simulink model "stepper_control"  (R2022a)
settings: Solver=FixedStepAuto  StartTime=0.0  StopTime=inf  FixedStep=0.00005  RelTol=1e-3
libraries: arduinolib x18, simulink x8, robotcorelib x2
settings Model: FPTRunName=Active  ExtModeTrigDuration=2  Creator=The MathWorks, Inc.  LastModifiedBy=15031
settings SolverCC: AlgebraicLoopSolver=TrustRegion
settings DataIOCC: LimitDataPoints=on  ReturnWorkspaceOutputs=off
settings OptimizationCC: ExpressionDepthLimit=2147483647  LifeSpan=Inf  MaxStackSize=64
settings DebuggingCC: UnderspecifiedInitializationDetection=Classic  MergeDetectMultiDrivingBlocksExec=none  FcnCallInpInsideContextMsg=warning  UnconnectedInputMsg=warning  UnconnectedOutputMsg=warning  UnconnectedLineMsg=warning  AllowSymbolicDim=off  StateNameClashWarn=warning  SFUnexpectedBacktrackingDiag=warning  SFNoUnconditionalDefaultTransitionDiag=warning  SFExecutionAtInitializationDiag=none  SFMachineParentedDataDiag=warning  ArithmeticOperatorsInVariantConditions=warning
settings HardwareCC: ProdBitPerInt=16  ProdBitPerPointer=16  ProdBitPerSizeT=16  ProdBitPerPtrDiffT=16  ProdLargestAtomicFloat=None  ProdWordSize=8  ProdHWDeviceType=Atmel->AVR  UseEmbeddedCoderFeatures=off  UseSimulinkCoderFeatures=off
settings ModelReferenceCC: PropagateSignalLabelsOutOfModel=off
settings SFSimCC: SimUseLocalCustomCode=off  MATLABDynamicMemAlloc=off
settings RTWCC: SystemTargetFile=ert.tlc  HardwareBoard=Arduino Mega 2560  TemplateMakefile=ert_default_tmf  GenerateReport=on  RTWVerbose=off  RTWUseLocalCustomCode=off  Toolchain=Arduino AVR  BuildConfiguration=Faster Runs  LaunchReport=on  DLArmComputeVersion=19.05
settings CodeAppCC: ForceParamTrailComments=on  OperatorAnnotations=on  StateflowObjectComments=on  MATLABSourceComments=on
settings ERTTargetCC: MultiwordLength=2048  ERTCustomFileBanners=off  SupportContinuousTime=on  SupportNonInlinedSFcns=on  RemoveResetFunc=off  ModelStepFunctionPrototypeControlCompliant=off
settings ConfigComp: CovMetricSettings=dw  CovSaveCumulativeToWorkspaceVar=on  CovSaveSingleToWorkspaceVar=on  CovExternalEMLEnable=off  CovSFcnEnable=off

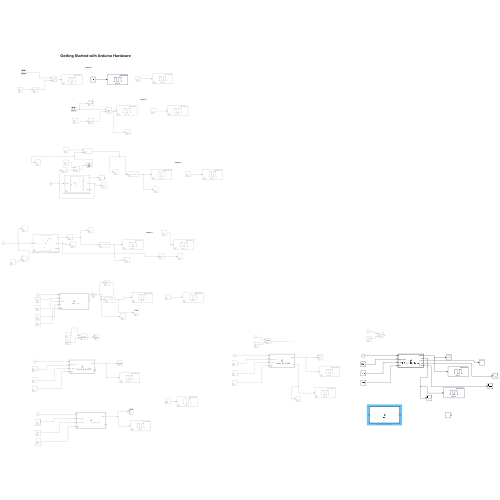
[thumbnail: Simulink's stored preview of the top-level diagram]
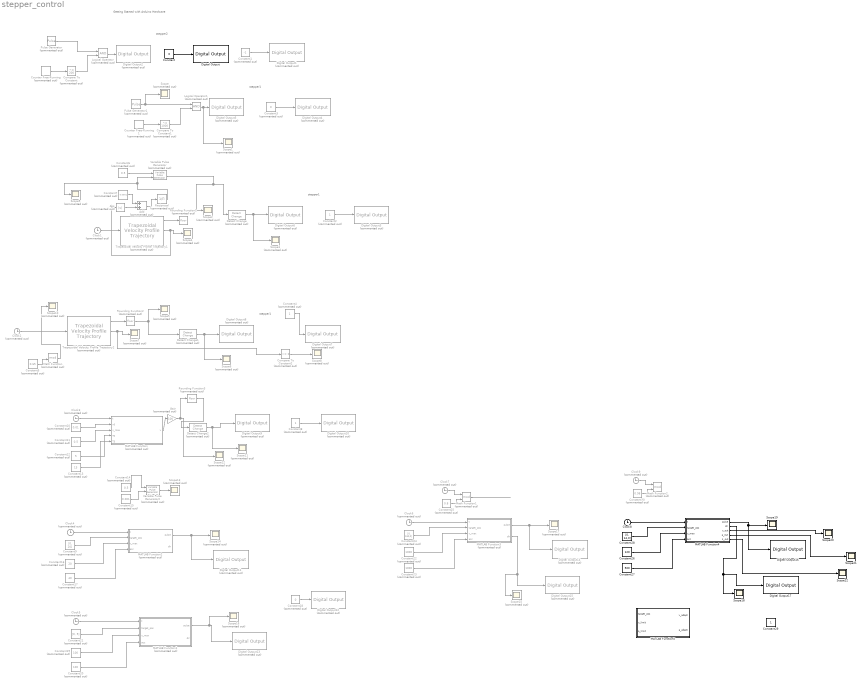
== system stepper_control ==
  note: stepper2
  note: Getting Started with Arduino Hardware
  note: stepper1
  note: stepper1
  note: stepper1
  Abs : Abs  Commented=on  SaturateOnIntegerOverflow=off
  Add : Sum  Commented=on
  Clock{1..7,9} (8 alike) : Clock  Commented=on
  Clock8 : Clock
  Compare To Constant : simulink/Logic and Bit Operations/Compare To Constant  Commented=on  relop=<=  const=200  OutDataTypeStr=boolean
  Compare To Constant1 : simulink/Logic and Bit Operations/Compare To Constant  Commented=on  relop=<=  const=1000  OutDataTypeStr=boolean
  Compare To Constant2 : simulink/Logic and Bit Operations/Compare To Constant  Commented=on  relop=>=  const=0  OutDataTypeStr=uint8
  Constant : Constant  Value=0
  Constant1 : Constant  Commented=on  Value=-1
  Constant10 : Constant  Commented=on  Value=0.01
  Constant11 : Constant  Commented=on  Value=0.5
  Constant12 : Constant  Commented=on  Value=5
  Constant13 : Constant  Commented=on  Value=13
  Constant14 : Constant  Commented=on  Value=0.5
  Constant15 : Constant  Commented=on  Value=0.001
  Constant16 : Constant  Commented=on  Value=20
  Constant17 : Constant  Commented=on  Value=40
  Constant18 : Constant  Commented=on  Value=0
  Constant19 : Constant  Commented=on  Value=100
  Constant2 : Constant  Commented=on
  Constant20 : Constant  Commented=on  Value=100
  Constant21 : Constant  Commented=on  Value=[0, 5]
  Constant22 : Constant  Commented=on  Value=1000
  Constant23 : Constant  Commented=on  Value=1000
  Constant24 : Constant  Commented=on  Value=[0, 240,0]
  Constant25 : Constant  Commented=on  Value=0.8
  Constant26 : Constant  Value=120
  Constant27 : Constant  Value=500
  Constant28 : Constant  Value=[0, 14,0]
  Constant29 : Constant
  Constant3 : Constant  Commented=on  Value=0
  Constant30 : Constant  Commented=on  Value=0.98
  Constant4 : Constant  Commented=on
  Constant5 : Constant  Commented=on  Value=0.65
  Constant6 : Constant  Commented=on  Value=0.5
  Constant7 : Constant  Commented=on  Value=0.0001
  Constant8 : Constant  Commented=on
  Constant9 : Constant  Commented=on  Value=[0, 20]
  Counter Free-Running : simulink/Sources/Counter Free-Running  Commented=on  NumBits=32  tsamp=0.002
  Counter Free-Running1 : simulink/Sources/Counter Free-Running  Commented=on  NumBits=32  tsamp=0.0002
  Detect Change : simulink/Logic and Bit Operations/Detect Change  Commented=on  vinit=0  OutDataTypeStr=uint8
  Detect Change1 : simulink/Logic and Bit Operations/Detect Change  Commented=on  vinit=0  InputProcessing=Columns as channels (frame based)  OutDataTypeStr=uint8
  Detect Change2 : simulink/Logic and Bit Operations/Detect Change  Commented=on  vinit=0  InputProcessing=Columns as channels (frame based)  OutDataTypeStr=uint8
  Digital Output : arduinolib/Digital Output  pinNumber=8  Direction=output  blockPlatform=arduino
  Digital Output{1,7,10,12} (4 alike) : arduinolib/Digital Output  Commented=on  pinNumber=6  Direction=output  blockPlatform=arduino
  Digital Output{2,8..9,11,13} (5 alike) : arduinolib/Digital Output  Commented=on  pinNumber=3  Direction=output  blockPlatform=arduino
  Digital Output14 : arduinolib/Digital Output  Commented=on  pinNumber=4  Direction=output  blockPlatform=arduino
  Digital Output15 : arduinolib/Digital Output  Commented=on  pinNumber=7  Direction=output  blockPlatform=arduino
  Digital Output16 : arduinolib/Digital Output  pinNumber=3  Direction=output  blockPlatform=arduino
  Digital Output17 : arduinolib/Digital Output  pinNumber=6  Direction=output  blockPlatform=arduino
  Digital Output3 : arduinolib/Digital Output  Commented=on  pinNumber=7  Direction=output  blockPlatform=arduino
  Digital Output4 : arduinolib/Digital Output  Commented=on  pinNumber=7  Direction=output  blockPlatform=arduino
  Digital Output5 : arduinolib/Digital Output  Commented=on  pinNumber=4  Direction=output  blockPlatform=arduino
  Digital Output6 : arduinolib/Digital Output  Commented=on  pinNumber=4  Direction=output  blockPlatform=arduino
  Gain : Gain  Commented=on  Gain=100
  Logical Operator : Logic  Commented=on  AllPortsSameDT=off  OutDataTypeStr=boolean
  Logical Operator1 : Logic  Commented=on  AllPortsSameDT=off  OutDataTypeStr=boolean
  MATLAB Function : MATLAB Function  Commented=on  TreatAsAtomicUnit=on
  MATLAB Function1 : MATLAB Function  Commented=on  TreatAsAtomicUnit=on
  MATLAB Function2 : MATLAB Function  Commented=on  TreatAsAtomicUnit=on
  MATLAB Function3 : MATLAB Function  Commented=on  TreatAsAtomicUnit=on
  MATLAB Function4 : MATLAB Function  TreatAsAtomicUnit=on
  MATLAB Function5 : MATLAB Function  TreatAsAtomicUnit=on
  Math Function : Math  Commented=on  Operator=mod
  Math Function1 : Math  Commented=on  Operator=mod
  Math Function2 : Math  Commented=on  Operator=mod
  Pulse Generator : DiscretePulseGenerator  Commented=on  SampleTime=0.001
  Pulse Generator1 : DiscretePulseGenerator  Commented=on  SampleTime=0.0001
  Reciprocal : Product  Commented=on  Inputs=/
  Rounding Function1 : Rounding  Commented=on
  Rounding Function2 : Rounding  Commented=on
  Rounding Function3 : Rounding  Commented=on
  Scope{,1..17} (18 alike) : Scope  Commented=on
  Scope{18..22} (5 alike) : Scope
  Trapezoidal Velocity Profile Trajectory1 : robotcorelib/Trapezoidal Velocity Profile Trajectory  Commented=on  WaypointSource=Internal  Waypoints=[0,2000]  NumParams=2  Parameter1=Acceleration  Parameter2=Peak Velocity  ParameterSource=Internal  PeakVelocity=5000  Acceleration=30000  EndTime=[ 1; 1 ]  AccelTime=[0,3 ]  SimulateUsing=Interpreted execution
      settings: SourceProductBaseCode=RO,NV,RR,UV
  Trapezoidal Velocity Profile Trajectory2 : robotcorelib/Trapezoidal Velocity Profile Trajectory  Commented=on  WaypointSource=Internal  Waypoints=[0,2300,0]  NumParams=2  Parameter1=Acceleration  Parameter2=Peak Velocity  ParameterSource=Internal  PeakVelocity=12000  Acceleration=100000  EndTime=[ 1; 1 ]  AccelTime=[0,3 ]  SimulateUsing=Interpreted execution
      settings: SourceProductBaseCode=RO,NV,RR,UV
  Variable Pulse Generator : VariablePulseGenerator  Commented=on  RunAtFixedTimeIntervals=on  SampleTime=0.0001
  Variable Pulse Generator2 : VariablePulseGenerator  Commented=on  AllowZeroPulseWidth=on  RunAtFixedTimeIntervals=on  SampleTime=0.00005
  wires:
  Pulse Generator/1 -> Logical Operator/1
  Constant/1 -> Digital Output/1
  Constant1/1 -> Digital Output1/1
  Compare To Constant/1 -> Logical Operator/2
  Logical Operator/1 -> Digital Output2/1
  Counter Free-Running/1 -> Compare To Constant/1
  Logical Operator1/1 -> Scope1/1, Digital Output5/1
  Pulse Generator1/1 -> Logical Operator1/1, Scope/1
  Counter Free-Running1/1 -> Compare To Constant1/1
  Compare To Constant1/1 -> Logical Operator1/2
  Constant3/1 -> Digital Output4/1
  Clock1/1 -> Trapezoidal Velocity Profile Trajectory1/1
  Constant2/1 -> Digital Output3/1
  Trapezoidal Velocity Profile Trajectory1/1 -> Rounding Function1/1
  Variable Pulse Generator/1 -> Scope2/1, Detect Change/1
  Trapezoidal Velocity Profile Trajectory1/2 -> Abs/1, Scope4/1
  Trapezoidal Velocity Profile Trajectory2/2 -> Compare To Constant2/1, Scope7/1
  Trapezoidal Velocity Profile Trajectory2/1 -> Rounding Function2/1
  Detect Change1/1 -> Scope6/1, Digital Output8/1
  Compare To Constant2/1 -> Scope8/1
  Rounding Function2/1 -> Scope5/1, Detect Change1/1
  Constant5/1 -> Math Function/2
  Detect Change/1 -> Scope3/1, Digital Output6/1
  Constant6/1 -> Variable Pulse Generator/1
  Abs/1 -> Add/2
  Reciprocal/1 -> Scope9/1, Variable Pulse Generator/2
  Add/1 -> Reciprocal/1
  Constant7/1 -> Add/1
  Clock2/1 -> Trapezoidal Velocity Profile Trajectory2/1
  Math Function/1 -> Scope10/1
  Clock3/1 -> MATLAB Function/1(t)
  Constant8/1 -> Digital Output10/1
  Constant10/1 -> MATLAB Function/2(v0)
  Constant11/1 -> MATLAB Function/3(v_max)
  Constant12/1 -> MATLAB Function/4(T0)
  Constant13/1 -> MATLAB Function/5(T3)
  Constant14/1 -> Variable Pulse Generator2/1
  Constant15/1 -> Variable Pulse Generator2/2
  Variable Pulse Generator2/1 -> Scope13/1
  Detect Change2/1 -> Scope11/1, Digital Output9/1
  MATLAB Function/1(v) -> Gain/1
  Gain/1 -> Rounding Function3/1, Scope12/1
  Rounding Function3/1 -> Detect Change2/1
  Constant17/1 -> MATLAB Function2/4(acc)
  Clock4/1 -> MATLAB Function2/1(t)
  Constant9/1 -> MATLAB Function2/2(target_pos)
  Constant16/1 -> MATLAB Function2/3(v_max)
  MATLAB Function2/1(pulse) -> Digital Output11/1, Scope14/1
  Constant4/1 -> Digital Output7/1
  Constant18/1 -> Digital Output12/1
  Constant21/1 -> MATLAB Function1/2(target_pos)
  Constant19/1 -> MATLAB Function1/3(v_max)
  Constant20/1 -> MATLAB Function1/4(acc)
  Clock5/1 -> MATLAB Function1/1(t)
  MATLAB Function1/1(pulse) -> Scope16/1, Digital Output13/1
  Constant24/1 -> MATLAB Function3/2(target_pos)
  Constant22/1 -> MATLAB Function3/3(v_max)
  MATLAB Function3/1(pulse) -> Digital Output14/1, Scope17/1
  Constant23/1 -> MATLAB Function3/4(acc)
  Clock6/1 -> MATLAB Function3/1(t)
  Constant25/1 -> Math Function1/2
  Math Function1/1 -> ?
  Clock7/1 -> Math Function1/1
  MATLAB Function3/2(dir) -> Digital Output15/1, Scope15/1
  Constant26/1 -> MATLAB Function4/3(v_max)
  Constant28/1 -> MATLAB Function4/2(target_pos)
  MATLAB Function4/2(dir) -> Scope18/1, Digital Output17/1
  MATLAB Function4/1(pulse) -> Digital Output16/1, Scope19/1
  Constant27/1 -> MATLAB Function4/4(acc)
  Constant30/1 -> Math Function2/2
  Clock9/1 -> Math Function2/1
  Clock8/1 -> MATLAB Function4/1(t)
  MATLAB Function4/3(v_out) -> Scope20/1
  MATLAB Function4/4(a_out) -> Scope21/1
  MATLAB Function4/5(s_out) -> Scope22/1

== matlab function stepper_control/MATLAB Function1 ==
  data: t input; pulse output; target_pos input; v_max input; acc input; dir output
function [pulse, dir] = S_Trapezoidal_Control(t, target_pos, v_max, acc)
    % 硬件常数定义 [cite: 73]
    K = 160; % 脉冲/mm [cite: 73]
    
    % 使用 persistent 变量存储状态，模仿单片机寄存器 [cite: 84, 125]
    persistent idx              % 当前目标点索引
    persistent startTime        % 当前路段起始时间
    persistent last_toggle_time % 上次脉冲翻转时间
    persistent current_state    % 当前脉冲电平状态
    
    % 初始化 [cite: 86]
    if isempty(idx)
        idx = 2; % 从 Waypoints 的第二个元素开始 (0 -> 2300)
        startTime = 0;
        last_toggle_time = 0;
        current_state = 0;
    end

    % --- 阶段 1: 轨迹规划与目标点切换 ---
    current_target = target_pos(idx);
    previous_target = target_pos(idx-1);
    S_total = abs(current_target - previous_target); % 本段总位移 [cite: 77]
    
    % 计算本段运行时间 (简化版 S-梯形时间分配) [cite: 23]
    % 注意：实际算法中 T0 需根据 S_total 校验，防止位移太短达不到 v_max [cite: 207]
    T_acc = 1.5 * (v_max / acc); % 加速阶段总长 [cite: 23, 210]
    T_const = S_total / v_max - T_acc; % 匀速阶段时长 [cite: 79]
    if T_const < 0, T_const = 0; end % 防错处理
    
    dt = t - startTime; % 本段已运行时间
    
    % 速度 v 计算 (根据论文公式 3 实现) [cite: 38, 72]
    T0 = v_max / (acc * 0.75); % 加加速特征时间 [cite: 23]
    if dt < T0
        v = 0.5 * (acc/T0) * dt^2; % 加加速 [cite: 31, 41]
    elseif dt < 1.5 * T0
        v = 0.5 * acc * T0 + acc * (dt - T0); % 匀加速 [cite: 36, 42]
    elseif dt < (1.5 * T0 + T_const)
        v = v_max; % 匀速 [cite: 32, 43]
    elseif dt < (3.0 * T0 + T_const)
        % 减速逻辑 (镜像加速过程) [cite: 23, 63]
        d_dt = (3.0 * T0 + T_const) - dt;
        v = 0.5 * (acc/T0) * d_dt^2;
    else
        v = 0;
        % 判定到达，切换到下一个路标点 
        if idx < length(target_pos)
            idx = idx + 1;
            startTime = t;
        end
    end

    % --- 阶段 2: 脉冲产生逻辑 --- [cite: 125]
    if v > 0.01
        T_pulse = 1 / (K * v); % 计算脉冲周期 [cite: 75]
        % 频率翻转逻辑 [cite: 102]
        if (t - last_toggle_time) >= (T_pulse / 2)
            current_state = 1 - current_state;
            last_toggle_time = t;
        end
    else
        current_state = 0;
    end

    % --- 阶段 3: 确定输出 (强制标量输出以防 Arduino 报错) ---
    pulse = double(current_state); % 必须是单个数值
    % 方向判定：根据当前目标与前一目标的差值确定 [cite: 21, 240]
    if current_target >= previous_target
        dir = 1.0; 
    else
        dir = 0.0;
    end
end

== matlab function stepper_control/MATLAB Function ==
  data: t input; v output; v0 input; v_max input; T0 input; T3 input
function v  = S_Curve_Gen(t, v0, v_max, T0, T3)
    % t: 当前仿真时间
    % v0: 启动速度
    % v_max: 设定运行速度 (Vh)
    % T0: 代数常数，用于确定加减速阶段时长 (根据论文 T_acc = 1.5*T0)
    % T3: 匀速阶段持续时间

    J = (v_max - v0) / (1.25 * T0^2); % 根据公式(3)推导的加加速度 J
    
    % 阶段时间节点定义 [cite: 23, 54]
    t1 = T0;               % 加加速结束
    t2 = 1.5 * T0;         % 匀加速结束（达到设定速度）
    t3 = t2 + T3;          % 匀速结束
    t4 = t3 + 0.5 * T0;    % 匀减速结束
    t5 = t3 + 1.5 * T0;    % 减减速结束（停止）

    if t >= 0 && t < t1
        % 加加速阶段 [cite: 31, 41]
        v = v0 + 0.5 * J * t^2;
    elseif t >= t1 && t < t2
        % 匀加速阶段 [cite: 36, 42]
        v = v0 - 0.5 * J * T0^2 + J * T0 * t;
    elseif t >= t2 && t < t3
        % 匀速阶段 [cite: 32, 43]
        v = v_max;
    elseif t >= t3 && t < t4
        % 匀减速阶段 [cite: 40, 44]
        v = v_max + 2.5 * J * T0^2 - J * T0 * (t - t3); % 参考公式(3)减速逻辑
    elseif t >= t4 && t <= t5
        % 减减速阶段 [cite: 69]
        % 此处根据公式(3)最后一段逻辑实现平滑减速至v0
        dt = t5 - t;
        v = v0 + 0.5 * J * dt^2;
    else
        v = 0; % 运行结束
    end
end

== matlab function stepper_control/MATLAB Function2 ==
  data: t input; pulse output; target_pos input; v_max input; acc input; dir output
function [pulse, dir] = S_Trapezoidal_Control(t, target_pos, v_max, acc)
    % 硬件常数：160 脉冲/mm
    K = 160; 
    
    % 持久变量：模拟单片机寄存器
    persistent idx startTime last_toggle_time current_state
    persistent T_acc T_const T_dec v_peak current_dist
    
    num_points = length(target_pos); 

    % 1. 初始化逻辑
    if isempty(idx)
        idx = 2; 
        startTime = 0;
        last_toggle_time = 0;
        current_state = 0;
        current_dist = 0; 
        
        % 初始化第一段参数
        p1 = target_pos(1);
        p2 = target_pos(min(idx, num_points));
        [T_acc, T_const, T_dec, v_peak] = calc_params(p1, p2, v_max, acc);
    end

    % 2. 确定当前参考点和总位移
    curr_idx = min(idx, num_points);
    prev_idx = max(1, curr_idx - 1);
    S_total = abs(target_pos(curr_idx) - target_pos(prev_idx)); 
    
    dt = t - startTime;
    T0 = v_peak / (acc * 0.75); % S曲线特征时间点 (加加速结束点)
    
    % 关键：定义完整的减速结束时间 T_end
    % S曲线对称性：加速耗时 1.5*T0, 减速耗时 1.5*T0
    T_end = 1.5*T0 + T_const + 1.5*T0;

    % --- 阶段 1: 速度规划与逻辑切换 ---
    if dt >= T_end || (current_dist >= S_total && S_total > 0 && dt > T_end*0.8)
        v = 0;
        % 到达终点，尝试切换到下一个路标
        if idx < num_points
            idx = idx + 1;
            startTime = t;
            current_dist = 0; 
            [T_acc, T_const, T_dec, v_peak] = calc_params(target_pos(idx-1), target_pos(idx), v_max, acc);
        end
    else
        % --- S-梯形速度分段函数 (核心修正) ---
        if dt < T0
            % 阶段1: 加加速 (速度按二次方上升)
            v = 0.5 * (acc/T0) * dt^2;
        elseif dt < 1.5 * T0
            % 阶段2: 匀加速 (速度线性上升)
            v = 0.5 * acc * T0 + acc * (dt - T0);
        elseif dt < (1.5 * T0 + T_const)
            % 阶段3: 匀速
            v = v_peak;
        elseif dt < (3.0 * T0 + T_const)
            % 阶段4: 减速 (镜像加速阶段，确保波形平滑变稀疏)
            % 计算距离终点的剩余时间 d_dt
            d_dt = (3.0 * T0 + T_const) - dt;
            if d_dt < 0, d_dt = 0; end
            v = 0.5 * (acc/T0) * d_dt^2; 
        else
            v = 0; 
        end
    end

    % --- 阶段 2: 脉冲翻转与位移累加 ---
    if v > 0.05
        T_period = 1 / (K * v); 
        if (t - last_toggle_time) >= (T_period / 2)
            current_state = 1 - current_state;
            last_toggle_time = t;
            % 仅在上升沿累加位移，保证精度
            if current_state == 1
                current_dist = current_dist + (1 / K);
            end
        end
    else
        current_state = 0;
    end

    % --- 阶段 3: 输出信号 ---
    pulse = double(current_state);
    if target_pos(curr_idx) >= target_pos(prev_idx)
        dir = 1.0; 
    else
        dir = 0.0;
    end
end

% 辅助函数：路段参数计算
function [Ta, Tc, Td, vp] = calc_params(p1, p2, vmax, a)
    dist = abs(p2 - p1);
    if dist < 1e-5, dist = 1e-5; end
    
    % 计算达到最大速度所需的最小距离 (S曲线加速+减速)
    S_acc_limit = 1.5 * (vmax^2 / a); 
    
    if dist >= S_acc_limit
        vp = vmax;
        Ta = 1.5 * (vmax / a);
        Tc = (dist - S_acc_limit) / vmax;
    else
        % 距离不足时，通过降速保证完整的S形起停
        vp = sqrt(dist * a / 1.5); 
        Ta = 1.5 * (vp / a);
        Tc = 0;
    end
    Td = Ta;
end

== matlab function stepper_control/MATLAB Function3 ==
  data: t input; pulse output; target_pos input; v_max input; acc input; dir output
function [pulse, dir] = S_Trapezoidal_Control(t, target_pos, v_max, acc)
    K = 160; % 160 pulses/mm
    persistent idx startTime last_toggle_time current_state current_dist
    persistent T_acc T_const v_peak
    
    num_pts = length(target_pos);
    if isempty(idx)
        idx = 2; startTime = 0; last_toggle_time = 0;
        current_state = 0; current_dist = 0;
        [T_acc, T_const, v_peak] = calc_logic(target_pos(1), target_pos(2), v_max, acc);
    end

    dt = t - startTime;
    S_total = abs(target_pos(idx) - target_pos(idx-1));
    T0 = v_peak / (acc * 0.75); 
    % 定义理论上的总耗时
    T_total = 3.0 * T0 + T_const; 

    % --- 修改后的阶段切换逻辑 ---
    % 只有当时间超过总时长，或者位移超标且速度极低时，才判定为到达
    if dt >= T_total || (current_dist >= S_total && dt > (T_total - T0))
        v = 0;
        if idx < num_pts
            idx = idx + 1; startTime = t; current_dist = 0;
            [T_acc, T_const, v_peak] = calc_logic(target_pos(idx-1), target_pos(idx), v_max, acc);
        end
    else
        % --- 速度规划逻辑 ---
        if dt < T0
            v = 0.5 * (acc/T0) * dt^2;
        elseif dt < 1.5 * T0
            v = 0.5 * acc * T0 + acc * (dt - T0);
        elseif dt < (1.5 * T0 + T_const)
            v = v_peak;
        elseif dt < T_total
            % 镜像减速：确保时间倒数到 T_total 时速度刚好为 0
            d_dt = T_total - dt;
            if d_dt < 0, d_dt = 0; end
            v = 0.5 * (acc/T0) * d_dt^2;
        else
            v = 0;
        end
    end

    % --- 脉冲产生 ---
    if v > 0.05
        T_p = 1 / (K * v);
        if (t - last_toggle_time) >= (T_p / 2)
            current_state = 1 - current_state;
            last_toggle_time = t;
            if current_state == 1, current_dist = current_dist + (1/K); end
        end
    else
        current_state = 0;
    end

    pulse = double(current_state);
    dir = double(target_pos(idx) >= target_pos(idx-1));
end

function [Ta, Tc, vp] = calc_logic(p1, p2, vmax, a)
    S = abs(p2 - p1);
    if S < 1e-4, S = 1e-4; end
    % S 曲线起停所需的最小距离
    S_limit = 1.5 * (vmax^2 / a); 
    
    if S >= S_limit
        vp = vmax;
        Ta = 1.5 * (vmax / a);
        Tc = (S - S_limit) / vmax;
    else
        % 自动降速，确保 S 曲线完整 (这是防止直接归零的关键)
        vp = sqrt(S * a / 1.5); 
        Ta = 1.5 * (vp / a);
        Tc = 0;
    end
end

== matlab function stepper_control/MATLAB Function4 ==
  data: t input; pulse output; target_pos input; v_max input; acc input; dir output; v_out output; a_out output; s_out output
function [pulse, dir, v_out, a_out, s_out] = S_Trapezoidal_Control(t, target_pos, v_max, acc)
    % 硬件常数：160 脉冲/mm
    K = 160; 
    
    persistent idx startTime last_toggle_time current_state current_dist
    persistent T_acc T_const v_peak
    
    num_pts = length(target_pos);
    if isempty(idx)
        idx = 2; startTime = 0; last_toggle_time = 0;
        current_state = 0; current_dist = 0;
        [T_acc, T_const, v_peak] = calc_logic(target_pos(1), target_pos(2), v_max, acc);
    end

    dt = t - startTime;
    S_segment = abs(target_pos(idx) - target_pos(idx-1)); % 当前段总路程
    T0 = v_peak / (acc * 0.75); 
    T_total = 3.0 * T0 + T_const; 

    v = 0; a = 0;

    % --- 阶段切换逻辑 ---
    if dt >= T_total || (current_dist >= S_segment && dt > (T_total - 0.5*T0))
        v = 0; a = 0;
        if idx < num_pts
            idx = idx + 1; startTime = t; current_dist = 0;
            [T_acc, T_const, v_peak] = calc_logic(target_pos(idx-1), target_pos(idx), v_max, acc);
        end
    else
        % --- 速度与加速度规划逻辑 (平滑衔接修正) ---
        if dt < T0
            v_raw = 0.5 * (acc/T0) * dt^2;
            v = min(v_raw, v_peak);
            a = (acc/T0) * dt; 
        elseif dt < 1.5 * T0
            v_raw = 0.5 * acc * T0 + acc * (dt - T0);
            if v_raw >= v_peak
                v = v_peak; a = 0;
            else
                v = v_raw; a = acc;
            end
        elseif dt < (1.5 * T0 + T_const)
            v = v_peak; a = 0;
        elseif dt < T_total
            d_dt = T_total - dt;
            if d_dt < 0, d_dt = 0; end
            if d_dt > T0
                v_raw = 0.5 * acc * T0 + acc * (d_dt - T0);
                a = -acc;
            else
                v_raw = 0.5 * (acc/T0) * d_dt^2;
                a = -(acc/T0) * d_dt;
            end
            v = min(v_raw, v_peak);
        else
            v = 0; a = 0;
        end
    end

    % --- 脉冲产生逻辑与路程物理累加 ---
    if v > 0.05
        T_p = 1 / (K * v);
        if (t - last_toggle_time) >= (T_p / 2)
            current_state = 1 - current_state;
            last_toggle_time = t;
            % 步进电机在脉冲上升沿移动 1/K mm
            if current_state == 1
                current_dist = current_dist + (1/K); 
            end
        end
    else
        current_state = 0;
    end

    % --- 输出赋值 ---
    pulse = double(current_state);
    dir = double(target_pos(idx) >= target_pos(idx-1));
    v_out = double(v); 
    a_out = double(a); 
    % s_out 输出当前路段已走过的累计位移
    s_out = double(current_dist); 
end

function [Ta, Tc, vp] = calc_logic(p1, p2, vmax, a)
    S = abs(p2 - p1);
    if S < 1e-4, S = 1e-4; end
    S_limit = 1.5 * (vmax^2 / a); 
    if S >= S_limit
        vp = vmax;
        Ta = 1.5 * (vmax / a);
        Tc = (S - S_limit) / vmax;
    else
        vp = sqrt(S * a / 1.5); 
        Ta = 1.5 * (vp / a);
        Tc = 0;
    end
end

== matlab function stepper_control/MATLAB Function5 ==
  data: target_pos input; v_adapt output; v_limit input; a_limit input; a_adapt output
function [v_adapt, a_adapt] = Parameter_Adapter(target_pos, v_limit, a_limit)
    % 输入：
    % target_pos: 目标位置点阵 [p1, p2, ...]
    % v_limit: 电机允许的极限最高速 (如 120)
    % a_limit: 电机允许的极限加速度 (如 1000)
    
    % 输出：
    % v_adapt, a_adapt: 为当前行程量身定制的 v 和 a
    
    % 1. 计算当前这一段的总行程
    if length(target_pos) < 2
        S = 0.01; % 极小值保护
    else
        S = abs(target_pos(2) - target_pos(1));
    end

    % 2. 距离敏感的自适应映射逻辑
    % 设定一些关键阈值
    S_threshold_micro = 5.0;  % 5mm 以下为微小行程
    S_threshold_long = 20.0;  % 20mm 以上为长行程

    if S < S_threshold_micro
        % 情况 A: 极短行程，大幅降速降加速，保证极致平稳
        % 速度随距离线性衰减，最小不低于 v_limit 的 20%
        v_ratio = max(0.2, S / S_threshold_micro);
        v_adapt = v_limit * v_ratio;
        a_adapt = a_limit * 0.5; % 加速度减半，防止震动
        
    elseif S < S_threshold_long
        % 情况 B: 中等行程，使用平方根映射保持 S 曲线形态
        % 这种映射方式能保证短行程也能跑出完整的“加-减”波形
        v_adapt = v_limit * sqrt(S / S_threshold_long);
        a_adapt = a_limit; % 使用标准加速度
        
    else
        % 情况 C: 长距离行程，全功率运行
        v_adapt = v_limit;
        a_adapt = a_limit;
    end
    
    % 3. 安全钳位 (Clamp)
    v_adapt = min(max(v_adapt, 5), v_limit); % 速度不低于 5mm/s，不高于极限
    a_adapt = min(max(a_adapt, 50), a_limit); % 加速度不低于 50mm/s^2
end
